simulink model "model_sim_CHBjt5"  (R2023b)
settings: Solver=FixedStepAuto  StartTime=0.0  StopTime=5  FixedStep=1e-6  RelTol=1e-3
InitFcn:
  | sysinit
StopFcn:
  | code_CHBJT5_stopfcn
values from neighbouring files (symbols this model uses):
  C = 0.0234    [sysinit.m]
  f = 50    [sysinit.m]
  f_switch = 250    [sysinit.m]
  fn = 50    [sysinit.m]
  L = 0.002    [sysinit.m]
  L_ori = 0.02    [sysinit.m]
  L_sec = 0.06    [sysinit.m]
  m = 0.95    [sysinit.m]
  P0 = 8e6    (= 8000000)    [sysinit.m]
  R = 1.5    [sysinit.m]
  Source_Amp = 10000    [sysinit.m]
  st = 1e-6    (= 1e-06)    [sysinit.m]
  Td = 15e-7    (= 1.5e-06)    [sysinit.m]
  Ts2 = 0.5e-3    (= 0.0005)    [sysinit.m]
  U_dcN = 2500    [sysinit.m]
  Ul_in = 1900    [sysinit.m]
undefined symbols (not defined in the file or in its folder): D1, Delta, magnitude
libraries: spsSeriesRLCBranchLib x63, spsDiodeLib x30, simulink x26, spsIGBTLib x24, spsMeanLib x20, spsCurrentMeasurementLib x10, spsThreePhaseVIMeasurementLib x7, spsOnDelayLib x6, spsUniversalBridgeLib x6, spsRMSLib x4, spsVoltageMeasurementLib x3, spsThreePhaseTransformerThreeWindingsLib x3
(part 2 of 2)

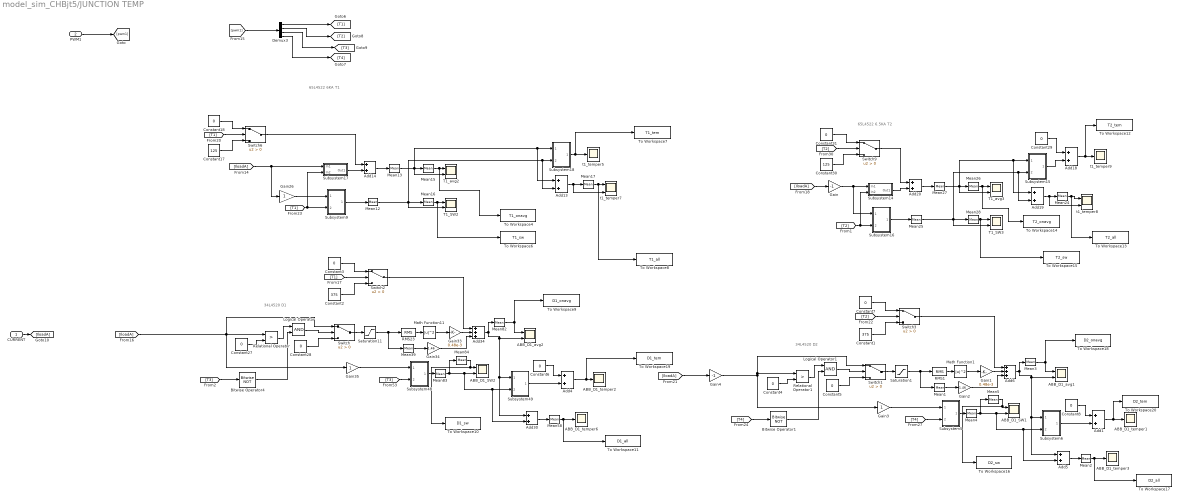
== system model_sim_CHBjt5/JUNCTION TEMP ==
  note: 65L4522 6.5KA T2
  note: 34L4520 D1
  note: 34L4520 D2
  note: 65L4522 6KA T1
  CURRENT : Inport
  PWM1 : Inport  Port=2
  ABB_D1_SW1 : Scope  NumInputPorts=2
  ABB_D1_SW2 : Scope  NumInputPorts=2
  ABB_D1_avg1 : Scope  NumInputPorts=2
  ABB_D1_avg2 : Scope  NumInputPorts=2
  ABB_D1_temper{1..3,6} (4 alike) : Scope
  Add{1,4..5,13..14,18..20,30} (9 alike) : Sum
  Add34 : Sum  Inputs=+++
  Add6 : Sum  Inputs=+++
  Bitwise Operator1 : simulink/Logic and Bit Operations/Bitwise Operator  logicop=NOT  UseBitMask=off  BitMask=bin2dec('11011001')  BitMaskRealWorld=Stored Integer
  Bitwise Operator4 : simulink/Logic and Bit Operations/Bitwise Operator  logicop=NOT  UseBitMask=off  BitMask=bin2dec('11011001')  BitMaskRealWorld=Stored Integer
  Constant1 : Constant  Value=375
  Constant17 : Constant  Value=125
  Constant{3..8,18,27..29,31} (11 alike) : Constant  Value=0
  Constant2 : Constant  Value=375
  Constant30 : Constant  Value=125
  Demux3 : Demux
  Gain : Gain  Gain=-1
  Gain1 : Gain  Gain=0.48e-3
  Gain2 : Gain  Gain=1.46
  Gain26 : Gain
  Gain3 : Gain
  Gain33 : Gain  Gain=0.48e-3
  Gain34 : Gain  Gain=1.46
  Gain35 : Gain
  Gain4 : Gain  Gain=-1
  Logical Operator : Logic  AllPortsSameDT=off  OutDataTypeStr=boolean
  Logical Operator1 : Logic  AllPortsSameDT=off  OutDataTypeStr=boolean
  Math Function1 : Math  Operator=magnitude^2  SignedPower=on
  Math Function11 : Math  Operator=magnitude^2  SignedPower=on
  Mean{1,4,12..13,25,27,39,83} (8 alike) : spsMeanLib/Mean  Freq=2000  Vinit=0  Ts=1e-6
  Mean{15..16,26,28} (4 alike) : spsMeanLib/Mean  Freq=f  Vinit=0  Ts=Ts2
  Mean{2..3,5,17,24,58,82,84} (8 alike) : spsMeanLib/Mean  Freq=f  Vinit=0  Ts=1e-6
  RMS1 : spsRMSLib/RMS  TrueRMS=on  Freq=2000  RMSInit=0  Ts=1e-6
  RMS23 : spsRMSLib/RMS  TrueRMS=on  Freq=2000  RMSInit=0  Ts=1e-6
  Relational Operator : RelationalOperator  Operator=>  OutDataTypeStr=boolean  RndMeth=Simplest  InputSameDT=off
  Relational Operator1 : RelationalOperator  Operator=>  OutDataTypeStr=boolean  RndMeth=Simplest  InputSameDT=off
  Saturation1 : Saturate  UpperLimit=5500  LowerLimit=0
  Saturation11 : Saturate  UpperLimit=5500  LowerLimit=0
  Subsystem14 : Subsystem
  Subsystem15 : Subsystem
  Subsystem16 : Subsystem
  Subsystem17 : Subsystem
  Subsystem18 : Subsystem
  Subsystem48 : Subsystem
  Subsystem49 : Subsystem
  Subsystem5 : Subsystem
  Subsystem6 : Subsystem
  Subsystem9 : Subsystem
  Switch{,1..3,6,9} (6 alike) : Switch  Criteria=u2 > Threshold  SaturateOnIntegerOverflow=off  InputSameDT=off
  T1_SW2 : Scope  NumInputPorts=2
  T1_SW3 : Scope  NumInputPorts=2
  T1_avg2 : Scope  NumInputPorts=2
  T1_avg3 : Scope  NumInputPorts=2
  To Workspace10 : ToWorkspace  VariableName=D1_sw  SaveFormat=Structure With Time  SampleTime=-1
  To Workspace11 : ToWorkspace  VariableName=D1_all  SaveFormat=Structure With Time  SampleTime=-1
  To Workspace12 : ToWorkspace  VariableName=T2_tem  SaveFormat=Structure With Time  SampleTime=-1
  To Workspace13 : ToWorkspace  VariableName=T2_all  SaveFormat=Structure With Time  SampleTime=-1
  To Workspace14 : ToWorkspace  VariableName=T2_onavg  SaveFormat=Structure With Time  SampleTime=-1
  To Workspace15 : ToWorkspace  VariableName=T2_sw  SaveFormat=Structure With Time  SampleTime=-1
  To Workspace16 : ToWorkspace  VariableName=D2_sw  SaveFormat=Structure With Time  SampleTime=-1
  To Workspace17 : ToWorkspace  VariableName=D2_all  SaveFormat=Structure With Time  SampleTime=-1
  To Workspace18 : ToWorkspace  VariableName=D2_onavg  SaveFormat=Structure With Time  SampleTime=-1
  To Workspace19 : ToWorkspace  VariableName=D1_tem  SaveFormat=Structure With Time  SampleTime=-1
  To Workspace20 : ToWorkspace  VariableName=D2_tem  SaveFormat=Structure With Time  SampleTime=-1
  To Workspace4 : ToWorkspace  VariableName=T1_onavg  SaveFormat=Structure With Time  SampleTime=-1
  To Workspace6 : ToWorkspace  VariableName=T1_sw  SaveFormat=Structure With Time  SampleTime=-1
  To Workspace7 : ToWorkspace  VariableName=T1_tem  SaveFormat=Structure With Time  SampleTime=-1
  To Workspace8 : ToWorkspace  VariableName=T1_all  SaveFormat=Structure With Time  SampleTime=-1
  To Workspace9 : ToWorkspace  VariableName=D1_onavg  SaveFormat=Structure With Time  SampleTime=-1
  t1_temper5 : Scope
  t1_temper7 : Scope  NumInputPorts=2
  t1_temper8 : Scope  NumInputPorts=2
  t1_temper9 : Scope
  wires:
  Mean24/1 -> To Workspace13/1, t1_temper8/1
  Mean13/1 -> T1_avg2/2, Mean15/1, Subsystem18/1(In1), Add13/1
  Add1/1 -> To Workspace20/1, ABB_D1_temper1/1
  Add20/1 -> Mean27/1
  Constant18/1 -> Switch6/1
  [T2] -> Switch9/2
  RMS1/1 -> Math Function1/1
  [T1] -> Subsystem9/2(In2), Subsystem17/2(In2)
  Saturation1/1 -> RMS1/1, Mean1/1
  Mean17/1 -> To Workspace8/1, t1_temper7/1
  Demux3/2 -> [T2]
  Mean12/1 -> Subsystem18/2(In2), Add13/2, T1_SW2/2, Mean16/1
  Bitwise Operator1/1 -> Logical Operator1/2
  Add5/1 -> Mean2/1
  Mean84/1 -> To Workspace10/1, ABB_D1_SW2/1
  Demux3/3 -> [T3]
  RMS23/1 -> Math Function11/1
  Add6/1 -> Mean3/1, ABB_D1_avg1/2, Subsystem6/1(In1), Add5/1
  Mean3/1 -> To Workspace18/1, ABB_D1_avg1/1
  [T3] -> Subsystem48/2(In2)
  Mean58/1 -> ABB_D1_temper6/1, To Workspace11/1
  Bitwise Operator4/1 -> Logical Operator/2
  Logical Operator/1 -> Switch/2
  Constant8/1 -> Add1/1
  Add14/1 -> Mean13/1
  Subsystem6/1(Out1) -> Add1/2
  Mean27/1 -> T1_avg3/2, Mean26/1, Subsystem15/1(In1), Add19/1
  Gain35/1 -> Subsystem48/1(In1)
  Add34/1 -> Add30/1, Subsystem49/1(In1), ABB_D1_avg2/2, Mean82/1
  Constant3/1 -> Switch2/1
  Math Function1/1 -> Gain1/1
  Subsystem18/1(Out1) -> To Workspace7/1, t1_temper5/1
  Subsystem5/1(Out1) -> Mean4/1
  Mean5/1 -> ABB_D1_SW1/1, To Workspace16/1
  Constant27/1 -> Relational Operator/2
  Switch9/1 -> Add20/1
  Gain3/1 -> Subsystem5/1(In1)
  Switch6/1 -> Add14/1
  Constant5/1 -> Switch1/3
  Constant6/1 -> Add4/1
  Relational Operator1/1 -> Logical Operator1/1
  Constant1/1 -> Switch3/3
  [pwm1] -> Demux3/1
  Gain34/1 -> Add34/3
  Constant7/1 -> Switch3/1
  [T4] -> Subsystem5/2(In2)
  [IloadA] -> Gain/1
  Constant4/1 -> Relational Operator1/2
  [T2] -> Switch3/2
  Switch/1 -> Saturation11/1
  Demux3/1 -> [T1]
  Mean28/1 -> To Workspace15/1, T1_SW3/1
  Add19/1 -> t1_temper8/2, Mean24/1
  [IloadA] -> Gain4/1
  Add4/1 -> To Workspace19/1, ABB_D1_temper2/1
  Add18/1 -> To Workspace12/1, t1_temper9/1
  [IloadA] -> Gain26/1, Subsystem17/1(In1)
  Demux3/4 -> [T4]
  Subsystem14/1(Out1) -> Add20/2
  Gain1/1 -> Add6/2
  Subsystem9/1(Out1) -> Mean12/1
  Switch1/1 -> Saturation1/1
  Logical Operator1/1 -> Switch1/2
  Subsystem16/1(Out1) -> Mean25/1
  Subsystem17/1(Out1) -> Add14/2
  Relational Operator/1 -> Logical Operator/1
  [T2] -> Subsystem14/2(In2), Subsystem16/2(In2)
  Gain2/1 -> Add6/3
  Constant2/1 -> Switch2/3
  Constant31/1 -> Switch9/1
  Constant29/1 -> Add18/1
  Mean82/1 -> ABB_D1_avg2/1, To Workspace9/1
  [T1] -> Switch2/2
  Gain26/1 -> Subsystem9/1(In1)
  Constant30/1 -> Switch9/3
  Subsystem15/1(Out1) -> Add18/2
  Mean83/1 -> Mean84/1, Add30/2, Subsystem49/2(In2), ABB_D1_SW2/2
  Mean25/1 -> Subsystem15/2(In2), Add19/2, T1_SW3/2, Mean28/1
  Mean26/1 -> To Workspace14/1, T1_avg3/1
  Subsystem48/1(Out1) -> Mean83/1
  Constant28/1 -> Switch/3
  Math Function11/1 -> Gain33/1
  Switch2/1 -> Add34/1
  Switch3/1 -> Add6/1
  Mean4/1 -> ABB_D1_SW1/2, Subsystem6/2(In2), Add5/2, Mean5/1
  [T3] -> Bitwise Operator4/1
  Mean16/1 -> To Workspace6/1, T1_SW2/1
  Saturation11/1 -> Mean39/1, RMS23/1
  Mean15/1 -> To Workspace4/1, T1_avg2/1
  [IloadA] -> Switch/1, Gain35/1, Relational Operator/1
  Add30/1 -> Mean58/1
  Mean2/1 -> To Workspace17/1, ABB_D1_temper3/1
  Add13/1 -> t1_temper7/2, Mean17/1
  [T4] -> Bitwise Operator1/1
  Subsystem49/1(Out1) -> Add4/2
  Constant17/1 -> Switch6/3
  Gain33/1 -> Add34/2
  Mean39/1 -> Gain34/1
  Mean1/1 -> Gain2/1
  [T1] -> Switch6/2
  CURRENT/1 -> [IloadA]
  PWM1/1 -> [pwm1]
  Gain/1 -> Subsystem16/1(In1), Subsystem14/1(In1)
  Gain4/1 -> Relational Operator1/1, Switch1/1, Gain3/1

== system model_sim_CHBjt5/LOAD ==
  Series RLC Branch1 : spsSeriesRLCBranchLib/Series RLC Branch  LConnTagsString=__new0  RConnTagsString=__new0  BranchType=RL  Resistance=R  Inductance=L  SetiL0=off  InitialCurrent=0  Capacitance=1e-6  Setx0=off  InitialVoltage=0  Measurements=None
  Series RLC Branch2 : spsSeriesRLCBranchLib/Series RLC Branch  LConnTagsString=__new0  RConnTagsString=__new0  BranchType=RL  Resistance=R  Inductance=L  SetiL0=off  InitialCurrent=0  Capacitance=1e-6  Setx0=off  InitialVoltage=0  Measurements=None
  Series RLC Branch7 : spsSeriesRLCBranchLib/Series RLC Branch  LConnTagsString=__new0  RConnTagsString=__new0  BranchType=RL  Resistance=R  Inductance=L  SetiL0=off  InitialCurrent=0  Capacitance=1e-6  Setx0=off  InitialVoltage=0  Measurements=None
  A : PMIOPort  Side=Left
  B : PMIOPort  Port=2  Side=Left
  C : PMIOPort  Port=3  Side=Left
  connections:
  Series RLC Branch7/RConn1 -- Series RLC Branch2/RConn1 -- Series RLC Branch1/RConn1
  Series RLC Branch2/LConn1 -- C/RConn1
  Series RLC Branch7/LConn1 -- A/RConn1
  Series RLC Branch1/LConn1 -- B/RConn1

== system model_sim_CHBjt5/Subsystem ==
  Current Measurement : spsCurrentMeasurementLib/Current Measurement  PhasorSimulation=off  OutputType=Complex  PSBequivalent=0
  Voltage Measurement : spsVoltageMeasurementLib/Voltage Measurement  PhasorSimulation=off  OutputType=Complex  PSBequivalent=0
  + : PMIOPort  Side=Left
  - : PMIOPort  Port=2  Side=Left
  +OUT : PMIOPort  Port=3  Side=Right
  -OUT : PMIOPort  Port=4  Side=Right
  tag scope: Idc=global, Udc=global
  wires:
  Voltage Measurement/1 -> [Udc]
  Current Measurement/1 -> [Idc]
  connections:
  Voltage Measurement/LConn1 -- Current Measurement/LConn1 -- +/RConn1
  Voltage Measurement/LConn2 -- -OUT/RConn1 -- -/RConn1
  Current Measurement/RConn1 -- +OUT/RConn1

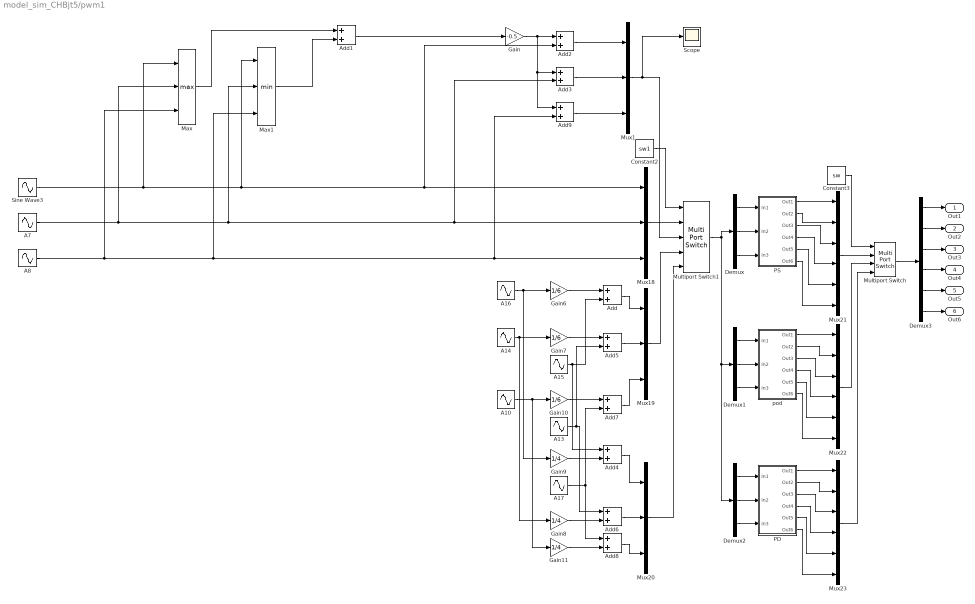
== system model_sim_CHBjt5/pwm1 ==
  A10 : Sin  Amplitude=m*1000  Frequency=2*pi*f*3  Phase=pi+2*pi/3  SampleTime=0
  A13 : Sin  Amplitude=m*1000  Frequency=2*pi*f  Phase=pi-2*pi/3  SampleTime=0
  A14 : Sin  Amplitude=m*1000  Frequency=2*pi*f*3  Phase=pi-2*pi/3  SampleTime=0
  A15 : Sin  Amplitude=m*1000  Frequency=2*pi*f  Phase=pi  SampleTime=0
  A16 : Sin  Amplitude=m*1000  Frequency=2*pi*f*3  Phase=pi  SampleTime=0
  A17 : Sin  Amplitude=m*1000  Frequency=2*pi*f  Phase=pi+2*pi/3  SampleTime=0
  A7 : Sin  Amplitude=m*1000  Frequency=2*pi*f  Phase=-2*pi/3  SampleTime=0
  A8 : Sin  Amplitude=m*1000  Frequency=2*pi*f  Phase=2*pi/3  SampleTime=0
  Add{,1..9} (10 alike) : Sum
  Constant2 : Constant  Value=sw1
  Constant3 : Constant  Value=sw
  Demux : Demux  Outputs=3
  Demux1 : Demux  Outputs=3
  Demux2 : Demux  Outputs=3
  Demux3 : Demux  Outputs=6
  Gain : Gain  Gain=-0.5
  Gain10 : Gain  Gain=1/6
  Gain11 : Gain  Gain=1/4
  Gain6 : Gain  Gain=1/6
  Gain7 : Gain  Gain=1/6
  Gain8 : Gain  Gain=1/4
  Gain9 : Gain  Gain=1/4
  Max : MinMax  Function=max  Inputs=3
  Max1 : MinMax  Inputs=3
  Multiport Switch : MultiPortSwitch  SaturateOnIntegerOverflow=off  InputSameDT=off
  Multiport Switch1 : MultiPortSwitch  Inputs=4  SaturateOnIntegerOverflow=off  InputSameDT=off
  Mux{1,18..20} (4 alike) : Mux  Inputs=3
  Mux21 : Mux  Inputs=6
  Mux22 : Mux  Inputs=6
  Mux23 : Mux  Inputs=6
  PD : Subsystem
  PS : Subsystem
  Scope : Scope
  Sine Wave3 : Sin  Amplitude=m*1000  Frequency=2*pi*f  SampleTime=0
  pod : Subsystem
  Out1 : Outport
  Out2 : Outport  Port=2
  Out3 : Outport  Port=3
  Out4 : Outport  Port=4
  Out5 : Outport  Port=5
  Out6 : Outport  Port=6
  wires:
  Gain8/1 -> Add6/2
  Demux3/2 -> Out2/1
  Demux1/1 -> pod/1(In1)
  Mux19/1 -> Multiport Switch1/4
  Demux3/6 -> Out6/1
  A10/1 -> Gain11/1, Gain10/1
  PD/1(Out1) -> Mux23/1
  PD/3(Out3) -> Mux23/3
  PD/2(Out2) -> Mux23/2
  Demux3/5 -> Out5/1
  PD/4(Out4) -> Mux23/4
  A13/1 -> Add5/2, Add6/1
  Demux2/1 -> PD/1(In1)
  Demux2/3 -> PD/3(In3)
  PD/5(Out5) -> Mux23/5
  PD/6(Out6) -> Mux23/6
  Add8/1 -> Mux20/3
  Add7/1 -> Mux19/3
  Add5/1 -> Mux19/2
  Add6/1 -> Mux20/2
  Constant2/1 -> Multiport Switch1/1
  PS/3(Out3) -> Mux21/3
  PS/4(Out4) -> Mux21/4
  PS/5(Out5) -> Mux21/5
  PS/2(Out2) -> Mux21/2
  Constant3/1 -> Multiport Switch/1
  Mux20/1 -> Multiport Switch1/5
  Gain10/1 -> Add7/1
  Gain7/1 -> Add5/1
  Mux21/1 -> Multiport Switch/2
  A8/1 -> Max/3, Max1/3, Add9/2, Mux18/3
  Gain9/1 -> Add4/2
  Gain6/1 -> Add/1
  Gain11/1 -> Add8/2
  Demux1/3 -> pod/3(In3)
  Demux1/2 -> pod/2(In2)
  Demux/3 -> PS/3(In3)
  Demux3/3 -> Out3/1
  Sine Wave3/1 -> Max/1, Max1/1, Add2/2, Mux18/1
  pod/4(Out4) -> Mux22/4
  pod/1(Out1) -> Mux22/1
  pod/3(Out3) -> Mux22/3
  pod/2(Out2) -> Mux22/2
  Demux3/4 -> Out4/1
  Multiport Switch/1 -> Demux3/1
  Demux2/2 -> PD/2(In2)
  Demux/1 -> PS/1(In1)
  Demux/2 -> PS/2(In2)
  pod/6(Out6) -> Mux22/6
  pod/5(Out5) -> Mux22/5
  PS/6(Out6) -> Mux21/6
  Demux3/1 -> Out1/1
  PS/1(Out1) -> Mux21/1
  Add/1 -> Mux19/1
  Add4/1 -> Mux20/1
  Multiport Switch1/1 -> Demux/1, Demux1/1, Demux2/1
  Mux18/1 -> Multiport Switch1/2
  Mux22/1 -> Multiport Switch/3
  Mux23/1 -> Multiport Switch/4
  A17/1 -> Add8/1, Add7/2
  A16/1 -> Gain9/1, Gain6/1
  A15/1 -> Add4/1, Add/2
  A14/1 -> Gain7/1, Gain8/1
  Max/1 -> Add1/1
  Max1/1 -> Add1/2
  Add1/1 -> Gain/1
  Gain/1 -> Add9/1, Add3/1, Add2/1
  Add9/1 -> Mux1/3
  Add3/1 -> Mux1/2
  Add2/1 -> Mux1/1
  A7/1 -> Max/2, Max1/2, Add3/2, Mux18/2
  Mux1/1 -> Scope/1, Multiport Switch1/3

== system model_sim_CHBjt5/3/-2//3*pi ==
  In1 : Inport
  Gain : Gain  Gain=-1
  Mux : Mux
  Mux1 : Mux
  NOT{,1..3} (4 alike) : Logic  Operator=NOT  AllPortsSameDT=off  OutDataTypeStr=boolean
  On Delay : spsOnDelayLib/On Delay  DelayType=On delay  delay=ttd  ic=0  Ts=0
  On Delay1 : spsOnDelayLib/On Delay  DelayType=On delay  delay=ttd  ic=0  Ts=0
  Relational Operator{,1..3} (4 alike) : RelationalOperator  Operator=>  OutDataTypeStr=boolean  RndMeth=Simplest  InputSameDT=off
  Repeating Sequence : simulink/Sources/Repeating Sequence  rep_seq_t=[0 0.5 1]/f_car  rep_seq_y=[-1 1 -1]*1000
  Transport Delay2 : TransportDelay  DelayTime=tt/f_car  BufferSize=3072
  Out1 : Outport
  Out2 : Outport  Port=2
  wires:
  On Delay1/1 -> Out2/1
  On Delay/1 -> Out1/1
  NOT/1 -> [S13]
  Transport Delay2/1 -> Relational Operator1/2, Relational Operator3/2
  [S14] -> Mux/4
  [S23] -> Mux1/3
  [S12] -> Mux/2
  In1/1 -> Gain/1, Relational Operator1/1, Relational Operator/1
  NOT2/1 -> [S14]
  [S21] -> Mux1/1
  Relational Operator1/1 -> NOT1/1, [S21]
  [S22] -> Mux1/2
  NOT3/1 -> [S24]
  Mux/1 -> On Delay/1
  Repeating Sequence/1 -> Relational Operator2/2, Relational Operator/2, Transport Delay2/1
  [S24] -> Mux1/4
  Gain/1 -> Relational Operator3/1, Relational Operator2/1
  [S13] -> Mux/3
  Relational Operator2/1 -> NOT2/1, [S12]
  [S11] -> Mux/1
  Relational Operator/1 -> NOT/1, [S11]
  NOT1/1 -> [S23]
  Mux1/1 -> On Delay1/1
  Relational Operator3/1 -> [S22], NOT3/1

== system model_sim_CHBjt5/3/0 ==
  In1 : Inport
  Gain : Gain  Gain=-1
  Mux : Mux
  Mux1 : Mux
  NOT{,1..3} (4 alike) : Logic  Operator=NOT  AllPortsSameDT=off  OutDataTypeStr=boolean
  On Delay1 : spsOnDelayLib/On Delay  DelayType=On delay  delay=ttd  ic=0  Ts=0
  On Delay2 : spsOnDelayLib/On Delay  DelayType=On delay  delay=ttd  ic=0  Ts=0
  Relational Operator{,1..3} (4 alike) : RelationalOperator  Operator=>  OutDataTypeStr=boolean  RndMeth=Simplest  InputSameDT=off
  Repeating Sequence : simulink/Sources/Repeating Sequence  rep_seq_t=[0 0.5 1]/f_car  rep_seq_y=[-1 1 -1]*1000
  Transport Delay2 : TransportDelay  DelayTime=tt/f_car  BufferSize=3072
  Out1 : Outport
  Out2 : Outport  Port=2
  wires:
  On Delay2/1 -> Out1/1
  On Delay1/1 -> Out2/1
  Relational Operator3/1 -> NOT3/1, [S22]
  Mux1/1 -> On Delay1/1
  NOT1/1 -> [S23]
  Relational Operator/1 -> [S11], NOT/1
  [S11] -> Mux/1
  Relational Operator2/1 -> [S12], NOT2/1
  [S13] -> Mux/3
  Gain/1 -> Relational Operator2/1, Relational Operator3/1
  [S24] -> Mux1/4
  Repeating Sequence/1 -> Transport Delay2/1, Relational Operator/2, Relational Operator2/2
  Mux/1 -> On Delay2/1
  NOT3/1 -> [S24]
  [S22] -> Mux1/2
  Relational Operator1/1 -> [S21], NOT1/1
  [S21] -> Mux1/1
  NOT2/1 -> [S14]
  In1/1 -> Relational Operator/1, Relational Operator1/1, Gain/1
  [S12] -> Mux/2
  [S23] -> Mux1/3
  [S14] -> Mux/4
  Transport Delay2/1 -> Relational Operator3/2, Relational Operator1/2
  NOT/1 -> [S13]

== system model_sim_CHBjt5/3/2//3*pi ==
  In1 : Inport
  Gain : Gain  Gain=-1
  Mux : Mux
  Mux1 : Mux
  NOT{,1..3} (4 alike) : Logic  Operator=NOT  AllPortsSameDT=off  OutDataTypeStr=boolean
  On Delay : spsOnDelayLib/On Delay  DelayType=On delay  delay=ttd  ic=0  Ts=0
  On Delay1 : spsOnDelayLib/On Delay  DelayType=On delay  delay=ttd  ic=0  Ts=0
  Relational Operator{,1..3} (4 alike) : RelationalOperator  Operator=>  OutDataTypeStr=boolean  RndMeth=Simplest  InputSameDT=off
  Repeating Sequence : simulink/Sources/Repeating Sequence  rep_seq_t=[0 0.5 1]/f_car  rep_seq_y=[-1 1 -1]*1000
  Transport Delay2 : TransportDelay  DelayTime=tt/f_car  BufferSize=3072
  Out1 : Outport
  Out2 : Outport  Port=2
  wires:
  On Delay1/1 -> Out2/1
  On Delay/1 -> Out1/1
  Relational Operator3/1 -> NOT3/1, [S22]
  Mux1/1 -> On Delay1/1
  NOT1/1 -> [S23]
  Relational Operator/1 -> [S11], NOT/1
  [S11] -> Mux/1
  Relational Operator2/1 -> [S12], NOT2/1
  [S13] -> Mux/3
  Gain/1 -> Relational Operator2/1, Relational Operator3/1
  [S24] -> Mux1/4
  Repeating Sequence/1 -> Transport Delay2/1, Relational Operator/2, Relational Operator2/2
  Mux/1 -> On Delay/1
  NOT3/1 -> [S24]
  [S22] -> Mux1/2
  Relational Operator1/1 -> [S21], NOT1/1
  [S21] -> Mux1/1
  NOT2/1 -> [S14]
  In1/1 -> Relational Operator/1, Relational Operator1/1, Gain/1
  [S12] -> Mux/2
  [S23] -> Mux1/3
  [S14] -> Mux/4
  Transport Delay2/1 -> Relational Operator3/2, Relational Operator1/2
  NOT/1 -> [S13]

== system model_sim_CHBjt5/3/Subsystem ==
  In1 : Inport
  In2 : Inport  Port=2
  In3 : Inport  Port=3
  Add{1..3,9} (4 alike) : Sum
  Gain : Gain  Gain=-0.5
  Max : MinMax  Function=max  Inputs=3
  Max1 : MinMax  Inputs=3
  Out1 : Outport
  Out2 : Outport  Port=2
  Out3 : Outport  Port=3
  wires:
  Add3/1 -> Out2/1
  Add2/1 -> Out1/1
  Add9/1 -> Out3/1
  Add1/1 -> Gain/1
  Max1/1 -> Add1/2
  Max/1 -> Add1/1
  Gain/1 -> Add2/1, Add3/1, Add9/1
  In1/1 -> Max/1, Add2/2, Max1/1
  In3/1 -> Max/3, Max1/3, Add9/2
  In2/1 -> Max/2, Max1/2, Add3/2

== system model_sim_CHBjt5/JUNCTION TEMP/Subsystem14 ==
  In1 : Inport
  In2 : Inport  Port=2
  Add : Sum
  Constant : Constant  Value=0
  Constant1 : Constant  Value=0
  Gain1 : Gain  Gain=0.39e-3
  Gain2 : Gain  Gain=1.39
  Gain3 : Gain
  Logical Operator : Logic  AllPortsSameDT=off  OutDataTypeStr=boolean
  Math Function : Math  Operator=magnitude^2  SignedPower=on
  Relational Operator : RelationalOperator  Operator=>  OutDataTypeStr=boolean  RndMeth=Simplest  InputSameDT=off
  Switch13 : Switch  Criteria=u2 > Threshold  SaturateOnIntegerOverflow=off  InputSameDT=off
  t1_temper{1..4} (4 alike) : Scope
  Out1 : Outport  VectorParamsAs1DForOutWhenUnconnected=off
  wires:
  Add/1 -> t1_temper4/1, Switch13/1
  Gain2/1 -> Add/2
  Math Function/1 -> Gain1/1
  In1/1 -> t1_temper3/1, Relational Operator/1, Gain3/1
  Gain1/1 -> Add/1
  Gain3/1 -> Gain2/1, Math Function/1
  Constant/1 -> Relational Operator/2
  Relational Operator/1 -> Logical Operator/1
  In2/1 -> t1_temper1/1, Logical Operator/2
  Logical Operator/1 -> t1_temper2/1, Switch13/2
  Switch13/1 -> Out1/1
  Constant1/1 -> Switch13/3

== system model_sim_CHBjt5/JUNCTION TEMP/Subsystem15 ==
  In1 : Inport
  In2 : Inport  Port=2
  Add1 : Sum  Inputs=5
  Add2 : Sum  Inputs=+++
  Add3 : Sum
  Constant1 : Constant  Value=40
  Discrete Filter1 : DiscreteFilter  Numerator=[Ts2/0.3]  Denominator=[1 (Ts2/0.3)-1]  SampleTime=Ts2
  Discrete Filter5 : DiscreteFilter  Numerator=[Ts2/605e-3]  Denominator=[1 (Ts2/605e-3)-1]  SampleTime=Ts2
  Discrete Filter6 : DiscreteFilter  Numerator=[Ts2/101e-3]  Denominator=[1 (Ts2/101e-3)-1]  SampleTime=Ts2
  Discrete Filter7 : DiscreteFilter  Numerator=[Ts2/5.2e-3]  Denominator=[1 (Ts2/5.2e-3)-1]  SampleTime=Ts2
  Discrete Filter8 : DiscreteFilter  Numerator=[Ts2/0.6e-3]  Denominator=[1 (Ts2/0.6e-3)-1]  SampleTime=Ts2
  Discrete Filter9 : DiscreteFilter  Numerator=[Ts2/0.5]  Denominator=[1 (Ts2/0.5)-1]  SampleTime=Ts2
  Gain1 : Gain  Gain=2.4e-3
  Gain5 : Gain  Gain=3.45e-3
  Gain6 : Gain  Gain=2.26e-3
  Gain7 : Gain  Gain=0.97e-3
  Gain8 : Gain  Gain=0.1e-3
  Gain9 : Gain  Gain=7.5e-3
  Out1 : Outport  VectorParamsAs1DForOutWhenUnconnected=off
  wires:
  In1/1 -> Add3/1
  In2/1 -> Add3/2
  Gain6/1 -> Discrete Filter6/1
  Gain9/1 -> Discrete Filter9/1
  Discrete Filter9/1 -> Add2/1
  Gain5/1 -> Discrete Filter5/1
  Discrete Filter6/1 -> Add1/2
  Gain7/1 -> Discrete Filter7/1
  Constant1/1 -> Add2/3
  Discrete Filter7/1 -> Add1/3
  Discrete Filter8/1 -> Add1/4
  Discrete Filter5/1 -> Add1/1
  Gain8/1 -> Discrete Filter8/1
  Add1/1 -> Add2/2
  Add2/1 -> Out1/1
  Discrete Filter1/1 -> Add1/5
  Gain1/1 -> Discrete Filter1/1
  Add3/1 -> Gain5/1, Gain9/1, Gain6/1, Gain7/1, Gain1/1, Gain8/1

== system model_sim_CHBjt5/JUNCTION TEMP/Subsystem16 ==
  In1 : Inport
  In2 : Inport  Port=2
  Abs1 : Abs  SaturateOnIntegerOverflow=off
  Add : Sum
  Constant1 : Constant  Value=0
  Constant2 : Constant  Value=0
  Gain1 : Gain  Gain=21.5/4000*U_dcN/2800
  Gain2 : Gain  Gain=3/4000*U_dcN/2800
  Gain3 : Gain  Gain=1/Ts2
  Gain4 : Gain
  Logical Operator : Logic  AllPortsSameDT=off  OutDataTypeStr=boolean
  Logical Operator1 : Logic  Operator=NOT  AllPortsSameDT=off  OutDataTypeStr=boolean
  Logical Operator2 : Logic  Operator=NOT  AllPortsSameDT=off  OutDataTypeStr=boolean
  Logical Operator3 : Logic  AllPortsSameDT=off  OutDataTypeStr=boolean
  Logical Operator4 : Logic  AllPortsSameDT=off  OutDataTypeStr=boolean
  Logical Operator5 : Logic  Operator=NOT  AllPortsSameDT=off  OutDataTypeStr=boolean
  Pulse Generator : DiscretePulseGenerator  PulseType=Time based  Period=Ts2  PulseWidth=5
  Scope1 : Scope  NumInputPorts=3
  Scope7 : Scope  NumInputPorts=2
  Switch{1..4} (4 alike) : Switch  Criteria=u2 > Threshold  SaturateOnIntegerOverflow=off  InputSameDT=off
  Unit Delay{,1..3} (4 alike) : UnitDelay  SampleTime=1e-6  HasFrameUpgradeWarning=on
  Out1 : Outport  VectorParamsAs1DForOutWhenUnconnected=off
  wires:
  In2/1 -> Logical Operator2/1, Logical Operator/1, Unit Delay/1
  Logical Operator/1 -> Switch1/2
  Abs1/1 -> Add/1
  Switch2/1 -> Gain1/1
  Switch1/1 -> Scope1/1, Abs1/1
  Unit Delay/1 -> Logical Operator3/1, Logical Operator1/1
  Logical Operator1/1 -> Logical Operator/2
  Logical Operator2/1 -> Logical Operator3/2
  Logical Operator3/1 -> Switch2/2
  Constant2/1 -> Switch2/3
  Gain2/1 -> Switch1/1
  Gain1/1 -> Switch1/3
  Switch3/1 -> Add/2
  Constant1/1 -> Switch3/1
  Pulse Generator/1 -> Unit Delay3/1, Logical Operator4/1
  Switch4/1 -> Scope7/2, Unit Delay2/1, Gain3/1
  Unit Delay2/1 -> Switch4/3
  Unit Delay3/1 -> Logical Operator5/1
  Logical Operator5/1 -> Logical Operator4/2
  Logical Operator4/1 -> Scope1/3, Switch4/2, Switch3/2
  Unit Delay1/1 -> Scope7/1, Switch3/3, Switch4/1
  Gain3/1 -> Out1/1
  In1/1 -> Gain4/1
  Add/1 -> Scope1/2, Unit Delay1/1
  Gain4/1 -> Switch2/1, Gain2/1

== system model_sim_CHBjt5/JUNCTION TEMP/Subsystem17 ==
  In1 : Inport
  In2 : Inport  Port=2
  Add : Sum
  Constant : Constant  Value=0
  Constant1 : Constant  Value=0
  Gain1 : Gain  Gain=0.39e-3
  Gain2 : Gain  Gain=1.39
  Gain3 : Gain
  Logical Operator : Logic  AllPortsSameDT=off  OutDataTypeStr=boolean
  Math Function : Math  Operator=magnitude^2  SignedPower=on
  Relational Operator : RelationalOperator  Operator=>  OutDataTypeStr=boolean  RndMeth=Simplest  InputSameDT=off
  Switch13 : Switch  Criteria=u2 > Threshold  SaturateOnIntegerOverflow=off  InputSameDT=off
  t1_temper{1..4} (4 alike) : Scope
  Out1 : Outport  VectorParamsAs1DForOutWhenUnconnected=off
  wires:
  Add/1 -> t1_temper4/1, Switch13/1
  Gain2/1 -> Add/2
  Math Function/1 -> Gain1/1
  In1/1 -> t1_temper3/1, Relational Operator/1, Gain3/1
  Gain1/1 -> Add/1
  Gain3/1 -> Gain2/1, Math Function/1
  Constant/1 -> Relational Operator/2
  Relational Operator/1 -> Logical Operator/1
  In2/1 -> t1_temper1/1, Logical Operator/2
  Logical Operator/1 -> t1_temper2/1, Switch13/2
  Switch13/1 -> Out1/1
  Constant1/1 -> Switch13/3

== system model_sim_CHBjt5/JUNCTION TEMP/Subsystem18 ==
  In1 : Inport
  In2 : Inport  Port=2
  Add1 : Sum  Inputs=5
  Add2 : Sum  Inputs=+++
  Add3 : Sum
  Constant1 : Constant  Value=40
  Discrete Filter1 : DiscreteFilter  Numerator=[Ts2/0.3]  Denominator=[1 (Ts2/0.3)-1]  SampleTime=Ts2
  Discrete Filter5 : DiscreteFilter  Numerator=[Ts2/605e-3]  Denominator=[1 (Ts2/605e-3)-1]  SampleTime=Ts2
  Discrete Filter6 : DiscreteFilter  Numerator=[Ts2/101e-3]  Denominator=[1 (Ts2/101e-3)-1]  SampleTime=Ts2
  Discrete Filter7 : DiscreteFilter  Numerator=[Ts2/5.2e-3]  Denominator=[1 (Ts2/5.2e-3)-1]  SampleTime=Ts2
  Discrete Filter8 : DiscreteFilter  Numerator=[Ts2/0.6e-3]  Denominator=[1 (Ts2/0.6e-3)-1]  SampleTime=Ts2
  Discrete Filter9 : DiscreteFilter  Numerator=[Ts2/0.5]  Denominator=[1 (Ts2/0.5)-1]  SampleTime=Ts2
  Gain1 : Gain  Gain=2.4e-3
  Gain5 : Gain  Gain=3.45e-3
  Gain6 : Gain  Gain=2.26e-3
  Gain7 : Gain  Gain=0.97e-3
  Gain8 : Gain  Gain=0.1e-3
  Gain9 : Gain  Gain=7.5e-3
  Out1 : Outport  VectorParamsAs1DForOutWhenUnconnected=off
  wires:
  In1/1 -> Add3/1
  In2/1 -> Add3/2
  Gain6/1 -> Discrete Filter6/1
  Gain9/1 -> Discrete Filter9/1
  Discrete Filter9/1 -> Add2/1
  Gain5/1 -> Discrete Filter5/1
  Discrete Filter6/1 -> Add1/2
  Gain7/1 -> Discrete Filter7/1
  Constant1/1 -> Add2/3
  Discrete Filter7/1 -> Add1/3
  Discrete Filter8/1 -> Add1/4
  Discrete Filter5/1 -> Add1/1
  Gain8/1 -> Discrete Filter8/1
  Add1/1 -> Add2/2
  Add2/1 -> Out1/1
  Discrete Filter1/1 -> Add1/5
  Gain1/1 -> Discrete Filter1/1
  Add3/1 -> Gain5/1, Gain9/1, Gain6/1, Gain7/1, Gain1/1, Gain8/1

== system model_sim_CHBjt5/JUNCTION TEMP/Subsystem48 ==
  In1 : Inport
  In2 : Inport  Port=2
  Abs1 : Abs  SaturateOnIntegerOverflow=off
  Add : Sum
  Constant1 : Constant  Value=0
  Constant2 : Constant  Value=0
  Fcn2 : Fcn  Expr=-2.8E-7*u*u+0.00278*u+3.056
  Gain1 : Gain  Gain=U_dcN/2800*11.5/13
  Gain2 : Gain  Gain=4.1/500
  Gain3 : Gain  Gain=1/Ts2
  Gain4 : Gain
  Logical Operator2 : Logic  Operator=NOT  AllPortsSameDT=off  OutDataTypeStr=boolean
  Logical Operator3 : Logic  AllPortsSameDT=off  OutDataTypeStr=boolean
  Logical Operator4 : Logic  AllPortsSameDT=off  OutDataTypeStr=boolean
  Logical Operator5 : Logic  Operator=NOT  AllPortsSameDT=off  OutDataTypeStr=boolean
  Pulse Generator : DiscretePulseGenerator  PulseType=Time based  Period=Ts2  PulseWidth=5
  Saturation : Saturate  UpperLimit=5500  LowerLimit=0
  Saturation1 : Saturate  UpperLimit=100  LowerLimit=0
  Scope1 : Scope  NumInputPorts=3
  Scope7 : Scope  NumInputPorts=2
  Switch1 : Switch  Criteria=u2 > Threshold  Threshold=500  SaturateOnIntegerOverflow=off  InputSameDT=off
  Switch2 : Switch  Criteria=u2 > Threshold  SaturateOnIntegerOverflow=off  InputSameDT=off
  Switch3 : Switch  Criteria=u2 > Threshold  SaturateOnIntegerOverflow=off  InputSameDT=off
  Switch4 : Switch  Criteria=u2 > Threshold  SaturateOnIntegerOverflow=off  InputSameDT=off
  Unit Delay{,1..3} (4 alike) : UnitDelay  SampleTime=1e-6  HasFrameUpgradeWarning=on
  Out1 : Outport  VectorParamsAs1DForOutWhenUnconnected=off
  wires:
  Abs1/1 -> Add/1
  Switch2/1 -> Gain1/1
  Gain1/1 -> Abs1/1, Scope1/1
  In2/1 -> Logical Operator3/1, Unit Delay/1
  Logical Operator2/1 -> Logical Operator3/2
  Logical Operator3/1 -> Switch2/2
  Constant2/1 -> Switch2/3
  Switch3/1 -> Add/2
  Constant1/1 -> Switch3/1
  Pulse Generator/1 -> Unit Delay3/1, Logical Operator4/1
  Switch4/1 -> Scope7/2, Unit Delay2/1, Gain3/1
  Unit Delay2/1 -> Switch4/3
  Unit Delay3/1 -> Logical Operator5/1
  Logical Operator5/1 -> Logical Operator4/2
  Logical Operator4/1 -> Scope1/3, Switch4/2, Switch3/2
  Unit Delay1/1 -> Scope7/1, Switch3/3, Switch4/1
  Gain3/1 -> Out1/1
  In1/1 -> Gain4/1
  Add/1 -> Scope1/2, Unit Delay1/1
  Unit Delay/1 -> Logical Operator2/1
  Fcn2/1 -> Switch1/1
  Gain4/1 -> Saturation/1
  Saturation/1 -> Fcn2/1, Switch1/2, Gain2/1
  Saturation1/1 -> Switch2/1
  Gain2/1 -> Switch1/3
  Switch1/1 -> Saturation1/1

== system model_sim_CHBjt5/JUNCTION TEMP/Subsystem49 ==
  In1 : Inport
  In2 : Inport  Port=2
  Add3 : Sum
  Add4 : Sum  Inputs=5
  Add5 : Sum  Inputs=+++
  Constant : Constant  Value=40
  Discrete Filter1 : DiscreteFilter  Numerator=[Ts2/5e-3]  Denominator=[1 (Ts2/5e-3)-1]  SampleTime=Ts2
  Discrete Filter2 : DiscreteFilter  Numerator=[Ts2/100e-3]  Denominator=[1 (Ts2/100e-3)-1]  SampleTime=Ts2
  Discrete Filter3 : DiscreteFilter  Numerator=[Ts2/800e-3]  Denominator=[1 (Ts2/800e-3)-1]  SampleTime=Ts2
  Discrete Filter4 : DiscreteFilter  Numerator=[Ts2/0.5]  Denominator=[1 (Ts2/0.5)-1]  SampleTime=Ts2
  Discrete Filter5 : DiscreteFilter  Numerator=[Ts2/300e-3]  Denominator=[1 (Ts2/300e-3)-1]  SampleTime=Ts2
  Gain1 : Gain  Gain=0.44e-3
  Gain2 : Gain  Gain=2.255e-3
  Gain3 : Gain  Gain=2.915e-3
  Gain4 : Gain  Gain=7.5e-3
  Gain5 : Gain  Gain=2.2e-3
  t1_temper : Scope
  t1_temper1 : Scope
  Out1 : Outport  VectorParamsAs1DForOutWhenUnconnected=off
  wires:
  In1/1 -> Add3/1
  Gain2/1 -> Discrete Filter2/1
  Discrete Filter2/1 -> Add4/3
  Discrete Filter3/1 -> Add4/4
  Add4/1 -> Add5/2
  Gain3/1 -> Discrete Filter3/1
  Add3/1 -> Gain5/1, t1_temper/1, Gain3/1, Gain4/1, Gain1/1, Gain2/1
  In2/1 -> Add3/2
  Constant/1 -> Add5/3
  Gain1/1 -> Discrete Filter1/1
  Gain4/1 -> Discrete Filter4/1
  Add5/1 -> Out1/1
  Discrete Filter1/1 -> Add4/2
  Discrete Filter4/1 -> t1_temper1/1, Add5/1
  Gain5/1 -> Discrete Filter5/1
  Discrete Filter5/1 -> Add4/5

== system model_sim_CHBjt5/JUNCTION TEMP/Subsystem5 ==
  In1 : Inport
  In2 : Inport  Port=2
  Abs1 : Abs  SaturateOnIntegerOverflow=off
  Add : Sum
  Constant1 : Constant  Value=0
  Constant2 : Constant  Value=0
  Fcn2 : Fcn  Expr=-2.8E-7*u*u+0.00278*u+3.056
  Gain1 : Gain  Gain=U_dcN/2800*11.5/13
  Gain2 : Gain  Gain=4.1/500
  Gain3 : Gain  Gain=1/Ts2
  Gain4 : Gain
  Logical Operator2 : Logic  Operator=NOT  AllPortsSameDT=off  OutDataTypeStr=boolean
  Logical Operator3 : Logic  AllPortsSameDT=off  OutDataTypeStr=boolean
  Logical Operator4 : Logic  AllPortsSameDT=off  OutDataTypeStr=boolean
  Logical Operator5 : Logic  Operator=NOT  AllPortsSameDT=off  OutDataTypeStr=boolean
  Pulse Generator : DiscretePulseGenerator  PulseType=Time based  Period=Ts2  PulseWidth=5
  Saturation : Saturate  UpperLimit=5500  LowerLimit=0
  Saturation1 : Saturate  UpperLimit=100  LowerLimit=0
  Scope1 : Scope  NumInputPorts=3
  Scope7 : Scope  NumInputPorts=2
  Switch1 : Switch  Criteria=u2 > Threshold  Threshold=500  SaturateOnIntegerOverflow=off  InputSameDT=off
  Switch2 : Switch  Criteria=u2 > Threshold  SaturateOnIntegerOverflow=off  InputSameDT=off
  Switch3 : Switch  Criteria=u2 > Threshold  SaturateOnIntegerOverflow=off  InputSameDT=off
  Switch4 : Switch  Criteria=u2 > Threshold  SaturateOnIntegerOverflow=off  InputSameDT=off
  Unit Delay{,1..3} (4 alike) : UnitDelay  SampleTime=1e-6  HasFrameUpgradeWarning=on
  Out1 : Outport  VectorParamsAs1DForOutWhenUnconnected=off
  wires:
  Switch1/1 -> Saturation1/1
  Gain2/1 -> Switch1/3
  Saturation1/1 -> Switch2/1
  Saturation/1 -> Gain2/1, Switch1/2, Fcn2/1
  Gain4/1 -> Saturation/1
  Fcn2/1 -> Switch1/1
  Unit Delay/1 -> Logical Operator2/1
  Add/1 -> Unit Delay1/1, Scope1/2
  In1/1 -> Gain4/1
  Gain3/1 -> Out1/1
  Unit Delay1/1 -> Switch4/1, Switch3/3, Scope7/1
  Logical Operator4/1 -> Switch3/2, Switch4/2, Scope1/3
  Logical Operator5/1 -> Logical Operator4/2
  Unit Delay3/1 -> Logical Operator5/1
  Unit Delay2/1 -> Switch4/3
  Switch4/1 -> Gain3/1, Unit Delay2/1, Scope7/2
  Pulse Generator/1 -> Logical Operator4/1, Unit Delay3/1
  Constant1/1 -> Switch3/1
  Switch3/1 -> Add/2
  Constant2/1 -> Switch2/3
  Logical Operator3/1 -> Switch2/2
  Logical Operator2/1 -> Logical Operator3/2
  In2/1 -> Unit Delay/1, Logical Operator3/1
  Gain1/1 -> Scope1/1, Abs1/1
  Switch2/1 -> Gain1/1
  Abs1/1 -> Add/1

== system model_sim_CHBjt5/JUNCTION TEMP/Subsystem6 ==
  In1 : Inport
  In2 : Inport  Port=2
  Add3 : Sum
  Add4 : Sum  Inputs=5
  Add5 : Sum  Inputs=+++
  Constant : Constant  Value=40
  Discrete Filter1 : DiscreteFilter  Numerator=[Ts2/5e-3]  Denominator=[1 (Ts2/5e-3)-1]  SampleTime=Ts2
  Discrete Filter2 : DiscreteFilter  Numerator=[Ts2/100e-3]  Denominator=[1 (Ts2/100e-3)-1]  SampleTime=Ts2
  Discrete Filter3 : DiscreteFilter  Numerator=[Ts2/800e-3]  Denominator=[1 (Ts2/800e-3)-1]  SampleTime=Ts2
  Discrete Filter4 : DiscreteFilter  Numerator=[Ts2/0.5]  Denominator=[1 (Ts2/0.5)-1]  SampleTime=Ts2
  Discrete Filter5 : DiscreteFilter  Numerator=[Ts2/300e-3]  Denominator=[1 (Ts2/300e-3)-1]  SampleTime=Ts2
  Gain1 : Gain  Gain=0.44e-3
  Gain2 : Gain  Gain=2.255e-3
  Gain3 : Gain  Gain=2.915e-3
  Gain4 : Gain  Gain=7.5e-3
  Gain5 : Gain  Gain=2.2e-3
  t1_temper : Scope
  t1_temper1 : Scope
  Out1 : Outport  VectorParamsAs1DForOutWhenUnconnected=off
  wires:
  Discrete Filter5/1 -> Add4/5
  Gain5/1 -> Discrete Filter5/1
  Discrete Filter4/1 -> Add5/1, t1_temper1/1
  Discrete Filter1/1 -> Add4/2
  Add5/1 -> Out1/1
  Gain4/1 -> Discrete Filter4/1
  Gain1/1 -> Discrete Filter1/1
  Constant/1 -> Add5/3
  In2/1 -> Add3/2
  Add3/1 -> Gain2/1, Gain1/1, Gain4/1, Gain3/1, t1_temper/1, Gain5/1
  Gain3/1 -> Discrete Filter3/1
  Add4/1 -> Add5/2
  Discrete Filter3/1 -> Add4/4
  Discrete Filter2/1 -> Add4/3
  Gain2/1 -> Discrete Filter2/1
  In1/1 -> Add3/1

== system model_sim_CHBjt5/JUNCTION TEMP/Subsystem9 ==
  In1 : Inport
  In2 : Inport  Port=2
  Abs1 : Abs  SaturateOnIntegerOverflow=off
  Add : Sum
  Constant1 : Constant  Value=0
  Constant2 : Constant  Value=0
  Gain1 : Gain  Gain=21.5/4000*U_dcN/2800
  Gain2 : Gain  Gain=3/4000*U_dcN/2800
  Gain3 : Gain  Gain=1/Ts2
  Gain4 : Gain
  Logical Operator : Logic  AllPortsSameDT=off  OutDataTypeStr=boolean
  Logical Operator1 : Logic  Operator=NOT  AllPortsSameDT=off  OutDataTypeStr=boolean
  Logical Operator2 : Logic  Operator=NOT  AllPortsSameDT=off  OutDataTypeStr=boolean
  Logical Operator3 : Logic  AllPortsSameDT=off  OutDataTypeStr=boolean
  Logical Operator4 : Logic  AllPortsSameDT=off  OutDataTypeStr=boolean
  Logical Operator5 : Logic  Operator=NOT  AllPortsSameDT=off  OutDataTypeStr=boolean
  Pulse Generator : DiscretePulseGenerator  PulseType=Time based  Period=Ts2  PulseWidth=5
  Scope1 : Scope  NumInputPorts=3
  Scope7 : Scope  NumInputPorts=2
  Switch{1..4} (4 alike) : Switch  Criteria=u2 > Threshold  SaturateOnIntegerOverflow=off  InputSameDT=off
  Unit Delay{,1..3} (4 alike) : UnitDelay  SampleTime=1e-6  HasFrameUpgradeWarning=on
  Out1 : Outport  VectorParamsAs1DForOutWhenUnconnected=off
  wires:
  In2/1 -> Logical Operator2/1, Logical Operator/1, Unit Delay/1
  Logical Operator/1 -> Switch1/2
  Abs1/1 -> Add/1
  Switch2/1 -> Gain1/1
  Switch1/1 -> Scope1/1, Abs1/1
  Unit Delay/1 -> Logical Operator3/1, Logical Operator1/1
  Logical Operator1/1 -> Logical Operator/2
  Logical Operator2/1 -> Logical Operator3/2
  Logical Operator3/1 -> Switch2/2
  Constant2/1 -> Switch2/3
  Gain2/1 -> Switch1/1
  Gain1/1 -> Switch1/3
  Switch3/1 -> Add/2
  Constant1/1 -> Switch3/1
  Pulse Generator/1 -> Unit Delay3/1, Logical Operator4/1
  Switch4/1 -> Scope7/2, Unit Delay2/1, Gain3/1
  Unit Delay2/1 -> Switch4/3
  Unit Delay3/1 -> Logical Operator5/1
  Logical Operator5/1 -> Logical Operator4/2
  Logical Operator4/1 -> Scope1/3, Switch4/2, Switch3/2
  Unit Delay1/1 -> Scope7/1, Switch3/3, Switch4/1
  Gain3/1 -> Out1/1
  In1/1 -> Gain4/1
  Add/1 -> Scope1/2, Unit Delay1/1
  Gain4/1 -> Switch2/1, Gain2/1

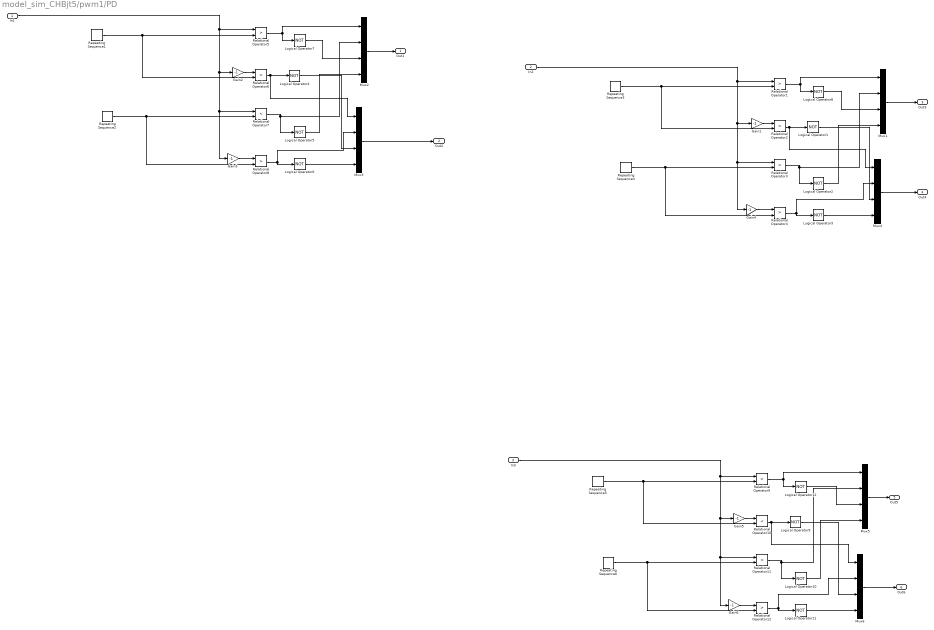
== system model_sim_CHBjt5/pwm1/PD ==
  In1 : Inport
  In2 : Inport  Port=2
  In3 : Inport  Port=3
  Gain{1..6} (6 alike) : Gain  Gain=-1
  Logical Operator{1..12} (12 alike) : Logic  Operator=NOT  AllPortsSameDT=off  OutDataTypeStr=boolean
  Mux{1..6} (6 alike) : Mux
  Relational Operator{1,4..5,8..9,12} (6 alike) : RelationalOperator  Operator=>  OutDataTypeStr=boolean  RndMeth=Simplest  InputSameDT=off
  Relational Operator{2..3,6..7,10..11} (6 alike) : RelationalOperator  Operator=<  OutDataTypeStr=boolean  RndMeth=Simplest  InputSameDT=off
  Repeating Sequence1 : simulink/Sources/Repeating Sequence  rep_seq_t=[0 0.5 1]/f_carrier  rep_seq_y=[0 1 0]*1000
  Repeating Sequence2 : simulink/Sources/Repeating Sequence  rep_seq_t=[0 0.5 1]/f_carrier  rep_seq_y=[-1 0 -1]*1000
  Repeating Sequence3 : simulink/Sources/Repeating Sequence  rep_seq_t=[0 0.5 1]/f_carrier  rep_seq_y=[0 1 0]*1000
  Repeating Sequence4 : simulink/Sources/Repeating Sequence  rep_seq_t=[0 0.5 1]/f_carrier  rep_seq_y=[-1 0 -1]*1000
  Repeating Sequence5 : simulink/Sources/Repeating Sequence  rep_seq_t=[0 0.5 1]/f_carrier  rep_seq_y=[0 1 0]*1000
  Repeating Sequence6 : simulink/Sources/Repeating Sequence  rep_seq_t=[0 0.5 1]/f_carrier  rep_seq_y=[-1 0 -1]*1000
  Out1 : Outport
  Out2 : Outport  Port=2
  Out3 : Outport  Port=3
  Out4 : Outport  Port=4
  Out5 : Outport  Port=5
  Out6 : Outport  Port=6
  wires:
  Logical Operator4/1 -> Mux3/3
  In1/1 -> Gain3/1, Relational Operator7/1, Gain2/1, Relational Operator5/1
  Relational Operator5/1 -> Logical Operator7/1, Mux2/1
  Gain2/1 -> Relational Operator6/1
  Repeating Sequence1/1 -> Relational Operator6/2, Relational Operator5/2
  Logical Operator7/1 -> Mux2/3
  Logical Operator6/1 -> Mux3/4
  Relational Operator6/1 -> Mux3/1, Logical Operator4/1
  Repeating Sequence2/1 -> Relational Operator8/2, Relational Operator7/2
  Mux3/1 -> Out2/1
  Relational Operator7/1 -> Mux2/2, Logical Operator5/1
  Logical Operator5/1 -> Mux2/4
  Relational Operator8/1 -> Mux3/2, Logical Operator6/1
  Gain3/1 -> Relational Operator8/1
  Mux2/1 -> Out1/1
  Logical Operator1/1 -> Mux4/3
  In2/1 -> Gain4/1, Relational Operator3/1, Gain1/1, Relational Operator1/1
  Relational Operator1/1 -> Logical Operator8/1, Mux1/1
  Gain1/1 -> Relational Operator2/1
  Repeating Sequence3/1 -> Relational Operator2/2, Relational Operator1/2
  Logical Operator8/1 -> Mux1/3
  Logical Operator3/1 -> Mux4/4
  Relational Operator2/1 -> Mux4/1, Logical Operator1/1
  Repeating Sequence4/1 -> Relational Operator4/2, Relational Operator3/2
  Relational Operator3/1 -> Mux1/2, Logical Operator2/1
  Logical Operator2/1 -> Mux1/4
  Relational Operator4/1 -> Mux4/2, Logical Operator3/1
  Gain4/1 -> Relational Operator4/1
  Mux4/1 -> Out4/1
  Mux1/1 -> Out3/1
  Logical Operator9/1 -> Mux6/3
  In3/1 -> Gain6/1, Relational Operator11/1, Gain5/1, Relational Operator9/1
  Relational Operator9/1 -> Logical Operator12/1, Mux5/1
  Gain5/1 -> Relational Operator10/1
  Repeating Sequence5/1 -> Relational Operator10/2, Relational Operator9/2
  Logical Operator12/1 -> Mux5/3
  Logical Operator11/1 -> Mux6/4
  Relational Operator10/1 -> Mux6/1, Logical Operator9/1
  Repeating Sequence6/1 -> Relational Operator12/2, Relational Operator11/2
  Mux6/1 -> Out6/1
  Relational Operator11/1 -> Mux5/2, Logical Operator10/1
  Logical Operator10/1 -> Mux5/4
  Relational Operator12/1 -> Mux6/2, Logical Operator11/1
  Gain6/1 -> Relational Operator12/1
  Mux5/1 -> Out5/1

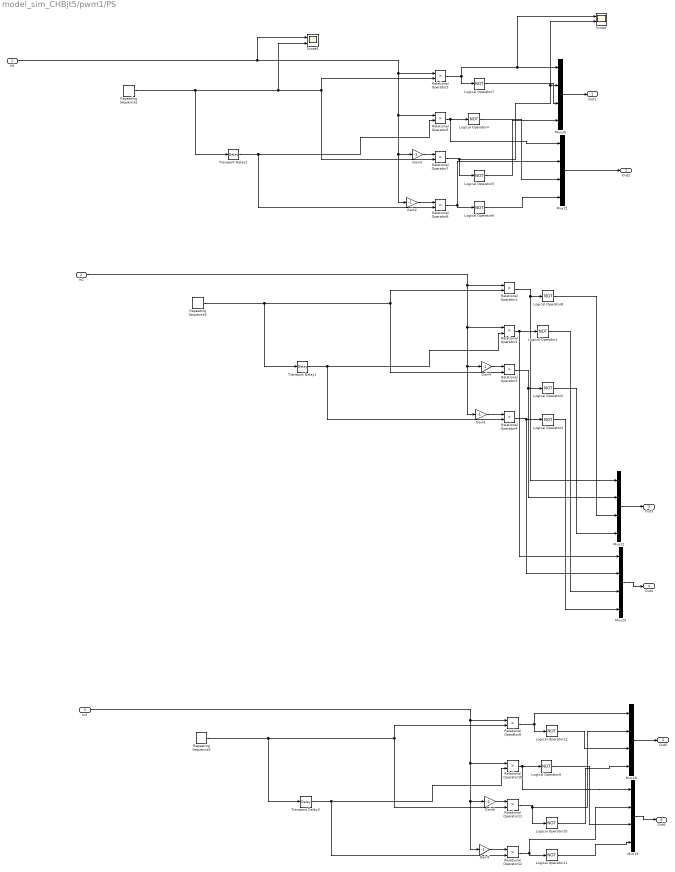
== system model_sim_CHBjt5/pwm1/PS ==
  In1 : Inport
  In2 : Inport  Port=2
  In3 : Inport  Port=3
  Gain{1..6} (6 alike) : Gain  Gain=-1
  Logical Operator{1..12} (12 alike) : Logic  Operator=NOT  AllPortsSameDT=off  OutDataTypeStr=boolean
  Mux{18..23} (6 alike) : Mux
  Relational Operator{1..12} (12 alike) : RelationalOperator  Operator=>  OutDataTypeStr=boolean  RndMeth=Simplest  InputSameDT=off
  Repeating Sequence1 : simulink/Sources/Repeating Sequence  rep_seq_t=[0 0.5 1]/f_carrier  rep_seq_y=[-1 1 -1]*1000
  Repeating Sequence2 : simulink/Sources/Repeating Sequence  rep_seq_t=[0 0.5 1]/f_carrier  rep_seq_y=[-1 1 -1]*1000
  Repeating Sequence3 : simulink/Sources/Repeating Sequence  rep_seq_t=[0 0.5 1]/f_carrier  rep_seq_y=[-1 1 -1]*1000
  Scope : Scope  NumInputPorts=2
  Scope1 : Scope  NumInputPorts=2
  Transport Delay1 : TransportDelay  DelayTime=0.25*(1/f_carrier)  BufferSize=3072
  Transport Delay2 : TransportDelay  DelayTime=0.25*(1/f_carrier)  BufferSize=3072
  Transport Delay3 : TransportDelay  DelayTime=0.25*(1/f_carrier)  BufferSize=3072
  Out1 : Outport
  Out2 : Outport  Port=2
  Out3 : Outport  Port=3
  Out4 : Outport  Port=4
  Out5 : Outport  Port=5
  Out6 : Outport  Port=6
  wires:
  Mux22/1 -> Out3/1
  Mux18/1 -> Out5/1
  Mux23/1 -> Out4/1
  Mux20/1 -> Out1/1
  Mux19/1 -> Out6/1
  Mux21/1 -> Out2/1
  Logical Operator6/1 -> Mux21/4
  In1/1 -> Scope1/1, Relational Operator6/1, Gain2/1, Gain3/1, Relational Operator5/1
  Logical Operator7/1 -> Mux20/3
  Logical Operator5/1 -> Mux20/4
  Relational Operator7/1 -> Mux20/2, Scope/2, Logical Operator5/1
  Relational Operator8/1 -> Mux21/2, Logical Operator6/1
  Transport Delay2/1 -> Relational Operator8/2, Relational Operator6/2
  Gain3/1 -> Relational Operator7/1
  Relational Operator6/1 -> Mux21/1, Logical Operator4/1
  Logical Operator4/1 -> Mux21/3
  Gain2/1 -> Relational Operator8/1
  Repeating Sequence1/1 -> Transport Delay2/1, Scope1/2, Relational Operator7/2, Relational Operator5/2
  Relational Operator5/1 -> Scope/1, Mux20/1, Logical Operator7/1
  Logical Operator3/1 -> Mux23/4
  In2/1 -> Relational Operator2/1, Gain1/1, Gain4/1, Relational Operator1/1
  Relational Operator3/1 -> Mux22/2, Logical Operator2/1
  Gain4/1 -> Relational Operator3/1
  Transport Delay1/1 -> Relational Operator4/2, Relational Operator2/2
  Relational Operator4/1 -> Mux23/2, Logical Operator3/1
  Logical Operator8/1 -> Mux22/3
  Logical Operator2/1 -> Mux22/4
  Logical Operator1/1 -> Mux23/3
  Relational Operator2/1 -> Mux23/1, Logical Operator1/1
  Gain1/1 -> Relational Operator4/1
  Repeating Sequence2/1 -> Transport Delay1/1, Relational Operator3/2, Relational Operator1/2
  Relational Operator1/1 -> Mux22/1, Logical Operator8/1
  Logical Operator11/1 -> Mux19/4
  In3/1 -> Relational Operator10/1, Gain5/1, Gain6/1, Relational Operator9/1
  Relational Operator11/1 -> Mux18/2, Logical Operator10/1
  Gain6/1 -> Relational Operator11/1
  Transport Delay3/1 -> Relational Operator12/2, Relational Operator10/2
  Relational Operator12/1 -> Mux19/2, Logical Operator11/1
  Logical Operator12/1 -> Mux18/3
  Logical Operator10/1 -> Mux18/4
  Logical Operator9/1 -> Mux19/3
  Relational Operator10/1 -> Mux19/1, Logical Operator9/1
  Gain5/1 -> Relational Operator12/1
  Repeating Sequence3/1 -> Transport Delay3/1, Relational Operator11/2, Relational Operator9/2
  Relational Operator9/1 -> Mux18/1, Logical Operator12/1

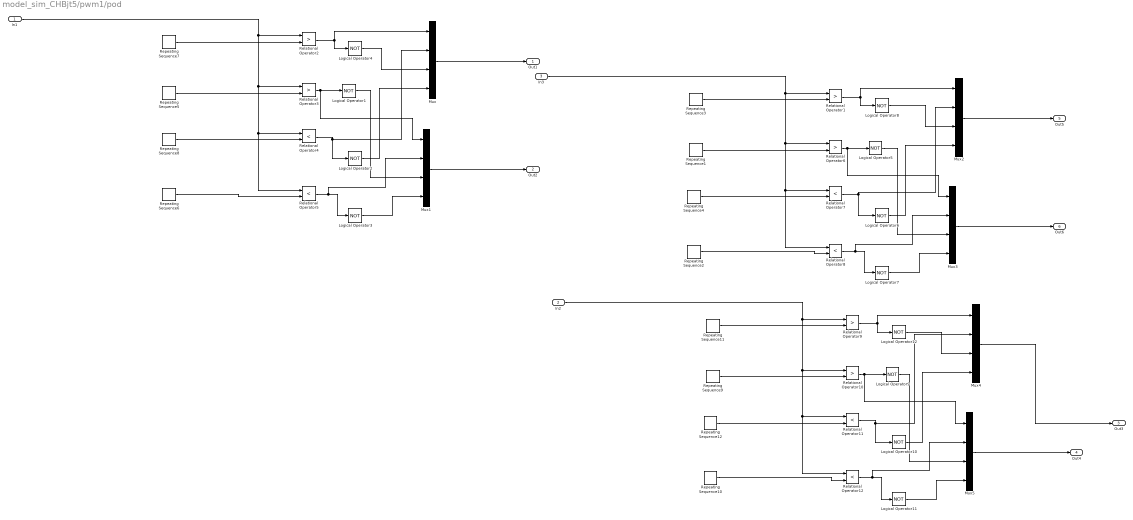
== system model_sim_CHBjt5/pwm1/pod ==
  In1 : Inport
  In2 : Inport  Port=2
  In3 : Inport  Port=3
  Logical Operator{1..12} (12 alike) : Logic  Operator=NOT  AllPortsSameDT=off  OutDataTypeStr=boolean
  Mux{,1..5} (6 alike) : Mux
  Relational Operator{1..3,6,9..10} (6 alike) : RelationalOperator  Operator=>  OutDataTypeStr=boolean  RndMeth=Simplest  InputSameDT=off
  Relational Operator{4..5,7..8,11..12} (6 alike) : RelationalOperator  Operator=<  OutDataTypeStr=boolean  RndMeth=Simplest  InputSameDT=off
  Repeating Sequence1 : simulink/Sources/Repeating Sequence  rep_seq_t=[0 0.5 1]*(1/f_carrier)  rep_seq_y=[0 1 0]*500
  Repeating Sequence10 : simulink/Sources/Repeating Sequence  rep_seq_t=[0 0.5 1]*(1/f_carrier)  rep_seq_y=[-2 -1 -2]*500
  Repeating Sequence11 : simulink/Sources/Repeating Sequence  rep_seq_t=[0 0.5 1]*(1/f_carrier)  rep_seq_y=[1 2 1]*500
  Repeating Sequence12 : simulink/Sources/Repeating Sequence  rep_seq_t=[0 0.5 1]*(1/f_carrier)  rep_seq_y=[-1 0 -1]*500
  Repeating Sequence2 : simulink/Sources/Repeating Sequence  rep_seq_t=[0 0.5 1]*(1/f_carrier)  rep_seq_y=[-2 -1 -2]*500
  Repeating Sequence3 : simulink/Sources/Repeating Sequence  rep_seq_t=[0 0.5 1]*(1/f_carrier)  rep_seq_y=[1 2 1]*500
  Repeating Sequence4 : simulink/Sources/Repeating Sequence  rep_seq_t=[0 0.5 1]*(1/f_carrier)  rep_seq_y=[-1 0 -1]*500
  Repeating Sequence5 : simulink/Sources/Repeating Sequence  rep_seq_t=[0 0.5 1]*(1/f_carrier)  rep_seq_y=[0 1 0]*500
  Repeating Sequence6 : simulink/Sources/Repeating Sequence  rep_seq_t=[0 0.5 1]*(1/f_carrier)  rep_seq_y=[-2 -1 -2]*500
  Repeating Sequence7 : simulink/Sources/Repeating Sequence  rep_seq_t=[0 0.5 1]*(1/f_carrier)  rep_seq_y=[1 2 1]*500
  Repeating Sequence8 : simulink/Sources/Repeating Sequence  rep_seq_t=[0 0.5 1]*(1/f_carrier)  rep_seq_y=[-1 0 -1]*500
  Repeating Sequence9 : simulink/Sources/Repeating Sequence  rep_seq_t=[0 0.5 1]*(1/f_carrier)  rep_seq_y=[0 1 0]*500
  Out1 : Outport
  Out2 : Outport  Port=2
  Out3 : Outport  Port=3
  Out4 : Outport  Port=4
  Out5 : Outport  Port=5
  Out6 : Outport  Port=6
  wires:
  Relational Operator3/1 -> Mux1/1, Logical Operator1/1
  Relational Operator5/1 -> Mux1/2, Logical Operator3/1
  Relational Operator4/1 -> Mux/2, Logical Operator2/1
  Mux1/1 -> Out2/1
  Logical Operator4/1 -> Mux/3
  Repeating Sequence7/1 -> Relational Operator2/2
  Logical Operator2/1 -> Mux/4
  Mux/1 -> Out1/1
  Relational Operator2/1 -> Logical Operator4/1, Mux/1
  Logical Operator3/1 -> Mux1/4
  In1/1 -> Relational Operator5/1, Relational Operator4/1, Relational Operator3/1, Relational Operator2/1
  Repeating Sequence5/1 -> Relational Operator3/2
  Logical Operator1/1 -> Mux1/3
  Logical Operator5/1 -> Mux3/3
  Repeating Sequence1/1 -> Relational Operator6/2
  In3/1 -> Relational Operator1/1, Relational Operator6/1, Relational Operator7/1, Relational Operator8/1
  Logical Operator7/1 -> Mux3/4
  Relational Operator1/1 -> Mux2/1, Logical Operator8/1
  Mux2/1 -> Out5/1
  Logical Operator6/1 -> Mux2/4
  Repeating Sequence2/1 -> Relational Operator8/2
  Repeating Sequence3/1 -> Relational Operator1/2
  Logical Operator8/1 -> Mux2/3
  Mux3/1 -> Out6/1
  Relational Operator7/1 -> Logical Operator6/1, Mux2/2
  Relational Operator8/1 -> Mux3/2, Logical Operator7/1
  Repeating Sequence4/1 -> Relational Operator7/2
  Relational Operator6/1 -> Logical Operator5/1, Mux3/1
  Relational Operator10/1 -> Mux5/1, Logical Operator9/1
  Repeating Sequence12/1 -> Relational Operator11/2
  Relational Operator12/1 -> Mux5/2, Logical Operator11/1
  Relational Operator11/1 -> Mux4/2, Logical Operator10/1
  Mux5/1 -> Out4/1
  Logical Operator12/1 -> Mux4/3
  Repeating Sequence11/1 -> Relational Operator9/2
  Repeating Sequence10/1 -> Relational Operator12/2
  Logical Operator10/1 -> Mux4/4
  Mux4/1 -> Out3/1
  Relational Operator9/1 -> Logical Operator12/1, Mux4/1
  Logical Operator11/1 -> Mux5/4
  In2/1 -> Relational Operator12/1, Relational Operator11/1, Relational Operator10/1, Relational Operator9/1
  Repeating Sequence9/1 -> Relational Operator10/2
  Logical Operator9/1 -> Mux5/3
  Repeating Sequence8/1 -> Relational Operator4/2
  Repeating Sequence6/1 -> Relational Operator5/2
